simulink model "TractorSprayerAndSensorModel3DSimulation"  (R2024b)
settings: Solver=VariableStepAuto  StartTime=0.0  StopTime=5  RelTol=1e-3
undefined symbols (not defined in the file): gray, refPosesT, refPosesX, refPosesY, sceneImage, Sim3dSensor
libraries: sim3dcameralib x1, sim3dautolib x1, sim3dlib x1
settings Model: Creator=sshenoy  LastModifiedBy=rhosea

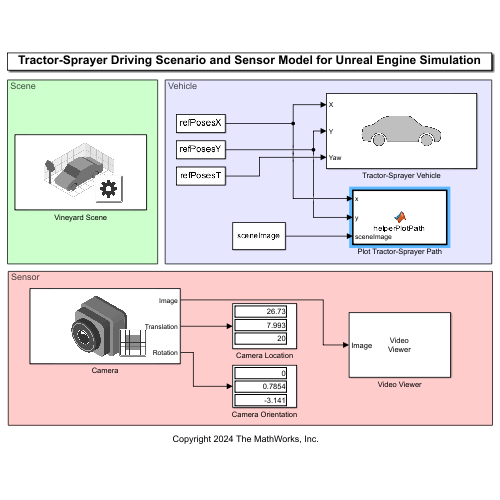
[thumbnail: Simulink's stored preview of the top-level diagram]
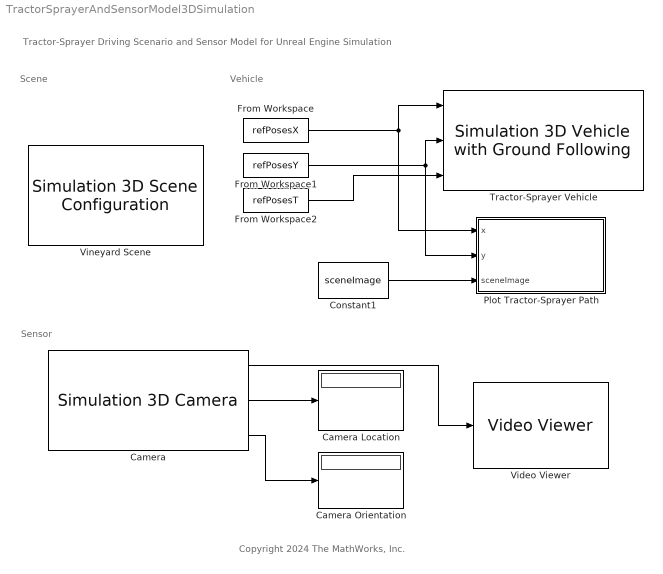
== system TractorSprayerAndSensorModel3DSimulation ==
  note: Scene
  note: Sensor
  note: Copyright 2024 The MathWorks, Inc.
  note: Tractor-Sprayer Driving Scenario and Sensor Model for Unreal Engine Simulation
  note: Vehicle
  Camera : sim3dcameralib/Simulation 3D Camera  Priority=1  sensorTag=Sim3dSensor�  sensorId=1  sensorName=Sim3dSensor�  vehTagList={'Scene Origin';'TractorSprayerVehicle'}  vehTag=TractorSprayerVehicle  mountLoc=Origin  offsetFlag=on  tmountOffset=[-20 0 20]  extTmount=off  rmountOffset=[0 45 0]  extRmount=off  FocalLength=[1109, 1109]  OpticalCenter=[640, 360]  ImageSize=[720, 1280]  RadialDistortion=[0, 0]  TangentialDistortion=[0, 0]  SensorSkew=0  DepthOutportEnabled=off  SemanticOutportEnabled=off  TransformOutportEnabled=on  SampleTime=-1  mountPoint=[-20 0 20]  mountOrientation=[0 -45 0]  aMode=6  ID=1
      settings: LibrarySourceBlock=robotsim3dlib/Simulation 3D Camera
  Camera Location : Display
  Camera Orientation : Display
  Constant1 : Constant  Value=sceneImage
  From Workspace : FromWorkspace  VariableName=refPosesX
  From Workspace1 : FromWorkspace  VariableName=refPosesY
  From Workspace2 : FromWorkspace  VariableName=refPosesT
  Plot Tractor-Sprayer Path : MATLAB Function  TreatAsAtomicUnit=on
  Tractor-Sprayer Vehicle : sim3dautolib/Simulation 3D Vehicle with Ground Following  Priority=1  PassVehMesh=Custom  MeshPath=/Game/Environment/Vehicles/TractorSprayer/TractorSprayer.TractorSprayer  TrackWidth=1.9  WheelBase=3  WheelRadius=0.35  VehColor=Red  InitialPos=[refPosesX(1,2), refPosesY(1,2),0]  InitialRot=[0, 0, refPosesT(1,2)]  ActorName=TractorSprayerVehicle  SampleTime=-1  ActorType=SimulinkVehicle  ID=C  aMode=5  ActorTag=TractorSprayerVehicle  CoordinateScheme=ISO  VehLightsControl=off  HeadlightColor=[ 1, 1, 1 ]  HighBeamIntensity=100000  LowBeamIntensity=60000  HighBeamConeAngle=70  LowBeamConeAngle=70  LeftHeadlightOrientation=[ 0, 0 ]  RightHeadlightOrientation=[ 0, 0 ]  BrakelightIntensity=500  ReverselightIntensity=500  SignallightIntensity=500  SignallightPeriod=1  SignalPulseWidth=50  TransformOutportEnabled=off
      settings: LibrarySourceBlock=sl3dlib/Simulation 3D/Actors/Simulation 3D Vehicle with Ground Following
  Video Viewer : VideoViewer  colormapValue=gray(256)  FigPos=[357 1006 565.333333333333 345.333333333333]
  Vineyard Scene : sim3dlib/Simulation 3D Scene Configuration  Priority=0  ProjectFormat=Unreal Executable  SceneDesc=Large parking lot  ProjectName=C:\Program Files\MATLAB\R2024b\toolbox\shared\sim3d_projects\automotive_project_windows\UE\WindowsNoEditor\VehicleSimulation.exe  ScenePath=/Game/Maps/Vineyard  UEProjPath=L:\UnrealWork\Bsim3d\scm\automotive_project_UE4\main\src\main\AutoVrtlEnv\AutoVrtlEnv.uproject  EnableOpenDRIVE=off  vehTagList={'Custom';'Scene Origin';'TractorSprayerVehicle'}  vehTag=TractorSprayerVehicle  FreeCameraInitialTranslation=[0, 0, 0]  FreeCameraDefaultInitialTranslation=[-6, 0, 2]  FreeCameraInitialRotation=[0, 0, 0]  FreeCameraDefaultInitialRotation=[0, -15, 0]  OpVisEn=off  Ts=1/60  EnableWindow=on  EnableRemoteAccess=off  EnableWeather=off  SunAzimuth=180.0  SunAltitude=0.0  EnableGeospatialSun=off  Latitude=0  Longitude=0  Date=2023-01-01  Time=10:30:00  GeoTimeZone=-5.0  SunDaylightSaving=off  wind=1  clouds=50.0  EnableVolumetricClouds=off  CloudCoverage=0  CloudAltitude=6  fog=0  rain=19.0  RaindropsEffect=off  SnowDensity=0  EnableGeospatial=off  UseTrueOrigin=off  OriginHeight=200  OriginLatitude=40.744652  OriginLongitude=-73.988864  MapStyle=Aerial  AdditionalAssetIDs=[]  UseAdvancedSunSky=off  SolarTime=11  TimeZone=-5  Day=21  Month=9  Year=2022  UseDaylightSavingTime=on  DSTStartDay=10  DSTStartMonth=3  DSTEndDay=3  DSTEndMonth=11  DSTSwitchHour=2  sensorTag=MainCamera1  sensorId=1  sensorName=MainCamera1  mountLoc=Origin  offsetFlag=off  tmountOffset=[0, 0, 0]  rmountOffset=[0, 0, 0]  HorizontalResolution=1280  VerticalResolution=720  HorizontalFOV=60  mountPoint=[0 0 0]  mountOrientation=[0 0 0]  aMode=3  ID=1  GeoTrigger=Inactive
      settings: LibrarySourceBlock=drivingsim3d/Simulation 3D Scene Configuration
  wires:
  Camera/2 -> Camera Location/1
  Camera/3 -> Camera Orientation/1
  Camera/1 -> Video Viewer/1
  From Workspace/1 -> Tractor-Sprayer Vehicle/1, Plot Tractor-Sprayer Path/1(x)
  From Workspace1/1 -> Plot Tractor-Sprayer Path/2(y), Tractor-Sprayer Vehicle/2
  From Workspace2/1 -> Tractor-Sprayer Vehicle/3
  Constant1/1 -> Plot Tractor-Sprayer Path/3(sceneImage)

== matlab function TractorSprayerAndSensorModel3DSimulation/Plot Tractor-Sprayer Path ==
  settings: updateMethod=DISCRETE
  data: x input; y input; sceneImage input
function helperPlotPath(x, y, sceneImage)
%helperPlotPath Plot path on scene image
%   helperPlotPath plots the path specified by x,y waypoint on the current
%   scene.

% Copyright 2019-2024 The MathWorks, Inc.

coder.extrinsic('helperShowVineyardSceneImage', 'helperShowSceneImage', ...
    'figure','movegui','isvalid','images.roi.Polyline',...
    'helperUpdatePolyline');

persistent hFig hPoly;

if isempty(hFig)
    
    % Create a figure and display the scene on it
    hFig = figure('Name', 'Scene Display');
    helperShowVineyardSceneImage(sceneImage);

    % Move figure to right of screen
    movegui(hFig, 'east')
    
    % Display the path
    hold on
    hPoly = images.roi.Polyline('Parent', gca, 'Position', [x y], 'InteractionsAllowed', 'none');
end

if isvalid(hFig)
    % Update the path with the new point
    helperUpdatePolyline(hPoly, x, y);
end
end
